simulink model "Myp5LinearOpenLoopObserver"  (R2021b)
settings: Solver=ode4  StartTime=0.0  StopTime=TIME_SIM  FixedStep=STEP_SIZE  RelTol=1e-3
values from neighbouring files (symbols this model uses):
  Aa = [-0.329723564087  0.00108308678514  -14.6666835708; 119.959269051  -1.23669349537  16746.7578957; 1  -0.0103092783505  0]    [LinearModel.mat]
  Bb = [-1.10657474768  0; 0  -0.0018722524695; 0  0]    [LinearModel.mat]
  Bv = [0.0209040137669 0 0]    [LinearModel.mat]
  Dd = [0  0; 0  0.0001229087]    [LinearModel.mat]
undefined symbols (not defined in the file or in its folder): Cc0, Ff, Gg, L, Ts
settings Model: Creator=tanzc  LastModifiedBy=tanzc
settings DataIOCC: SaveFormat=Array  ReturnWorkspaceOutputs=off

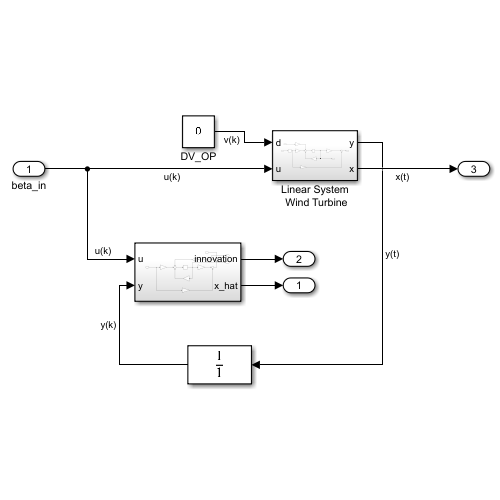
[thumbnail: Simulink's stored preview of the top-level diagram]
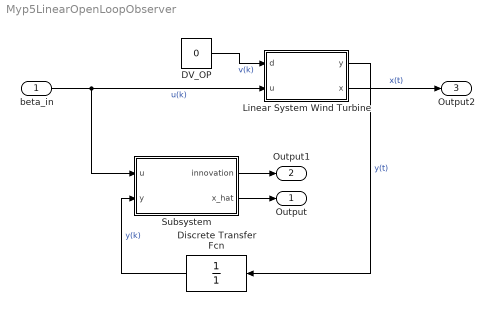
== system Myp5LinearOpenLoopObserver ==
  beta_in : Inport
  DV_OP : Constant  Value=0
  Discrete Transfer Fcn : DiscreteTransferFcn  Denominator=1  SampleTime=Ts
  Linear System Wind Turbine : Subsystem
  Subsystem : Subsystem
  Output : Outport
  Output1 : Outport  Port=2
  Output2 : Outport  Port=3
  wires:
  beta_in/1 -> Subsystem/1(u), Linear System Wind Turbine/2(u)  "u(k)"
  DV_OP/1 -> Linear System Wind Turbine/1(d)  "v(k)"
  Linear System Wind Turbine/1(y) -> Discrete Transfer Fcn/1  "y(t)"
  Linear System Wind Turbine/2(x) -> Output2/1  "x(t)"
  Discrete Transfer Fcn/1 -> Subsystem/2(y)  "y(k)"
  Subsystem/1(innovation) -> Output1/1
  Subsystem/2(x_hat) -> Output/1

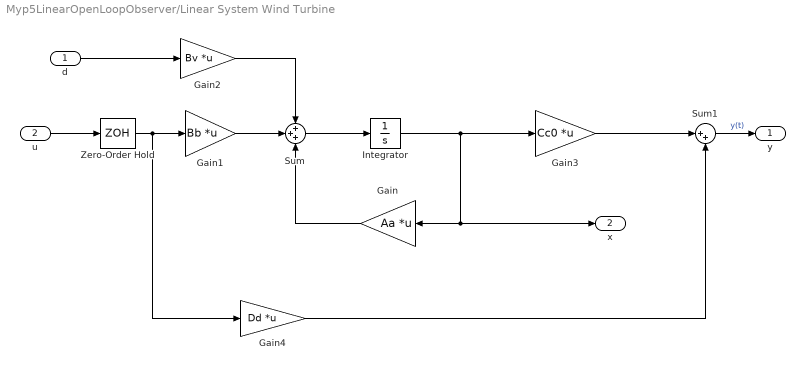
== system Myp5LinearOpenLoopObserver/Linear System Wind Turbine ==
  d : Inport
  u : Inport  Port=2
  Gain : Gain  Gain=Aa  Multiplication=Matrix(K*u) (u vector)
  Gain1 : Gain  Gain=Bb  Multiplication=Matrix(K*u) (u vector)
  Gain2 : Gain  Gain=Bv  Multiplication=Matrix(K*u) (u vector)
  Gain3 : Gain  Gain=Cc0  Multiplication=Matrix(K*u) (u vector)
  Gain4 : Gain  Gain=Dd  Multiplication=Matrix(K*u) (u vector)
  Integrator : Integrator
  Sum : Sum  Inputs=+++
  Sum1 : Sum  Inputs=|++
  Zero-Order Hold : ZeroOrderHold  SampleTime=Ts
  y : Outport
  x : Outport  Port=2
  wires:
  d/1 -> Gain2/1
  Integrator/1 -> Gain3/1, x/1, Gain/1
  Gain2/1 -> Sum/1
  Gain/1 -> Sum/3
  Gain1/1 -> Sum/2
  Sum/1 -> Integrator/1
  Zero-Order Hold/1 -> Gain4/1, Gain1/1
  u/1 -> Zero-Order Hold/1
  Gain3/1 -> Sum1/1
  Gain4/1 -> Sum1/2
  Sum1/1 -> y/1  "y(t)"

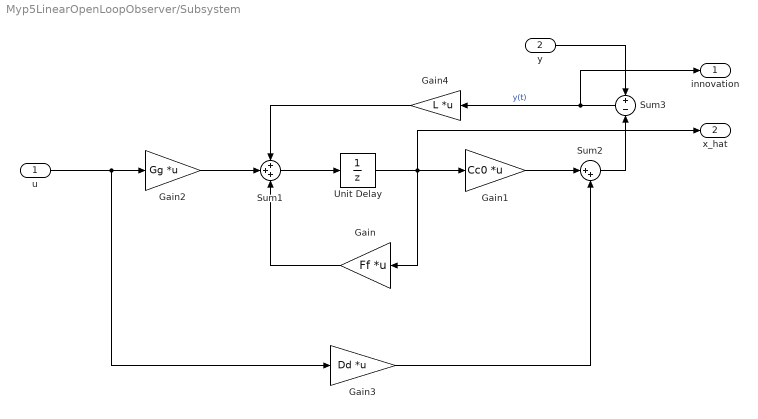
== system Myp5LinearOpenLoopObserver/Subsystem ==
  u : Inport
  y : Inport  Port=2
  Gain : Gain  Gain=Ff  Multiplication=Matrix(K*u) (u vector)
  Gain1 : Gain  Gain=Cc0  Multiplication=Matrix(K*u) (u vector)
  Gain2 : Gain  Gain=Gg  Multiplication=Matrix(K*u) (u vector)
  Gain3 : Gain  Gain=Dd  Multiplication=Matrix(K*u) (u vector)
  Gain4 : Gain  Gain=L  Multiplication=Matrix(K*u) (u vector)
  Sum1 : Sum  Inputs=+++
  Sum2 : Sum  Inputs=|++
  Sum3 : Sum  Inputs=+-
  Unit Delay : UnitDelay  SampleTime=Ts  HasFrameUpgradeWarning=on
  innovation : Outport
  x_hat : Outport  Port=2
  wires:
  y/1 -> Sum3/1
  Gain1/1 -> Sum2/1
  Unit Delay/1 -> x_hat/1, Gain/1, Gain1/1
  Gain2/1 -> Sum1/2
  Sum2/1 -> Sum3/2
  u/1 -> Gain3/1, Gain2/1
  Gain3/1 -> Sum2/2
  Gain/1 -> Sum1/3
  Gain4/1 -> Sum1/1
  Sum1/1 -> Unit Delay/1
  Sum3/1 -> innovation/1, Gain4/1  "y(t)"
